simulink model "continuos_model"  (R2016b)
settings: Solver=VariableStepAuto  StartTime=0.0  StopTime=40  FixedStep=0.001  RelTol=1e-3
undefined symbols (not defined in the file or in its folder): DiscIntNeverNeededParam
libraries: dspsrcs4 x2
settings Model: Creator=Utente  LastModifiedBy=liana

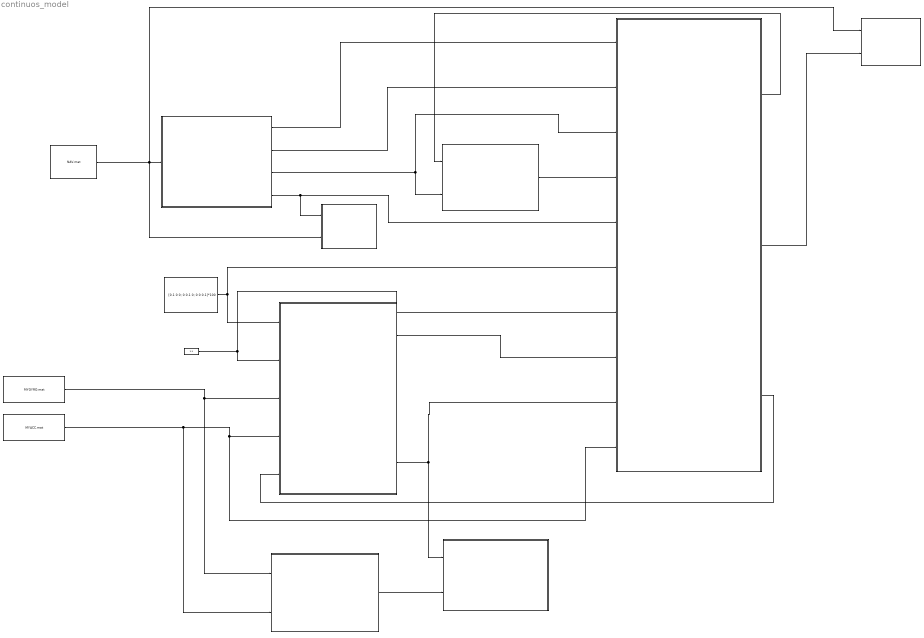
== system continuos_model ==
  Algebraic Transformation : Subsystem
  Attitude Observer : Subsystem
  Error position (AT) : Subsystem
  Error position (NLO) : Subsystem
  From File2 : FromFile  FileName=MYGYRO.mat
  From File3 : FromFile  FileName=MYACC.mat
  Gain computation : Subsystem
  Kp : Constant  Value=[0.1 0 0; 0 0.1 0; 0 0 0.1]*100  SampleTime=-1
  Mechanisation : Subsystem
  Translational Motion Observer : Subsystem
  Vehicle position in NED : FromFile  FileName=NAV.mat
  angles error : Subsystem
  sigma : Constant  Value=1.1  SampleTime=-1
  wires:
  From File2/1 -> Mechanisation/1(w_ib), Attitude Observer/3(w_ib)
  From File3/1 -> Mechanisation/2(f_b), Translational Motion Observer/10(f_b), Attitude Observer/4(f_b)
  Kp/1 -> Translational Motion Observer/6(K_p), Attitude Observer/1(Kp)
  sigma/1 -> Attitude Observer/2(sigma), Translational Motion Observer/7(sigma)
  Attitude Observer/1(J) -> Translational Motion Observer/8(J)
  Attitude Observer/3(R_nb_stim) -> Translational Motion Observer/9(R_nb_stim), angles error/1(R_nb_stim)
  Gain computation/1(K) -> Translational Motion Observer/4(K)
  Algebraic Transformation/3(C_dx) -> Translational Motion Observer/3(C_dx), Gain computation/2(C_dx)
  Translational Motion Observer/2(x_stim) -> Error position (NLO)/2(estimated)
  Vehicle position in NED/1 -> Error position (NLO)/1(true), Error position (AT)/2(true), Algebraic Transformation/1(p_n)
  Translational Motion Observer/3(f_n_stim) -> Attitude Observer/5(f_n_stim)
  Algebraic Transformation/4(x_at) -> Translational Motion Observer/5(Init), Error position (AT)/1(estimated)
  Mechanisation/1(R_nb) -> angles error/2(R_nb)
  Algebraic Transformation/1(p_n_i) -> Translational Motion Observer/1(p_n_i)
  Translational Motion Observer/1(C_dx_NLO) -> Gain computation/1(C_dx_NLO)
  Algebraic Transformation/2(delta) -> Translational Motion Observer/2(delta)

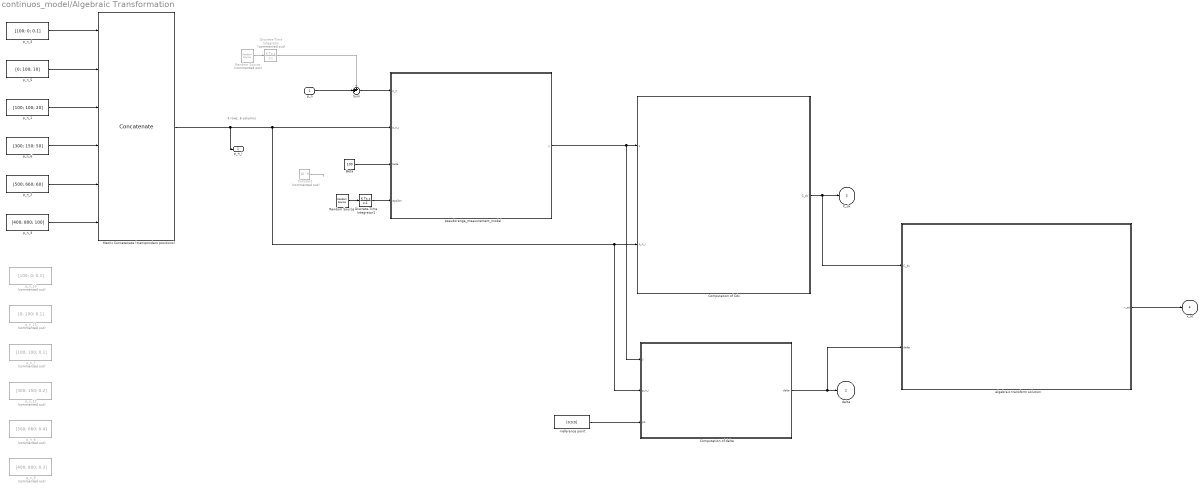
== system continuos_model/Algebraic Transformation ==
  note: 3 rows, 6 columns
  p_n : Inport
  Beta : Constant  Value=100  SampleTime=0.1
  Computation of Cdx : MATLAB Function  TreatAsAtomicUnit=on
  Computation of delta : MATLAB Function  TreatAsAtomicUnit=on
  Constant : Constant  Commented=on  Value=10^6
  Discrete-Time Integrator : DiscreteIntegrator  Commented=on  IntegratorMethod=Integration: Backward Euler  gainval=2  InitialConditionSetting=State (most efficient)  SampleTime=0.1  LimitOutput=on  UpperSaturationLimit=10  LowerSaturationLimit=-10  ICPrevOutput=DiscIntNeverNeededParam  ICPrevScaledInput=DiscIntNeverNeededParam
  Discrete-Time Integrator1 : DiscreteIntegrator  IntegratorMethod=Integration: Backward Euler  gainval=10  InitialConditionSetting=State (most efficient)  SampleTime=0.1  LimitOutput=on  UpperSaturationLimit=10  LowerSaturationLimit=-10  ICPrevOutput=DiscIntNeverNeededParam  ICPrevScaledInput=DiscIntNeverNeededParam
  Matrix Concatenate (transponders positions) : Concatenate  NumInputs=6  Mode=Multidimensional array  ConcatenateDimension=2
  Random Source : dspsrcs4/Random Source  Commented=on  SrcType=Gaussian  NormMethod=Ziggurat  CltLength=12  MinVal=0  MaxVal=1  MeanVal=[0;0;0]  VarVal=[1;1;1]*0.25  RepMode=Not repeatable  rawSeed=1  IsInherit=off  SampMode=Discrete  SampTime=0.1  SampFrame=1  DataType=Double  OutComplex=Real  OutputFrames=off
  Random Source1 : dspsrcs4/Random Source  SrcType=Gaussian  NormMethod=Ziggurat  CltLength=12  MinVal=0  MaxVal=1  MeanVal=0  VarVal=0.25  RepMode=Not repeatable  rawSeed=1  IsInherit=off  SampMode=Discrete  SampTime=0.1  SampFrame=1  DataType=Single  OutComplex=Real  OutputFrames=off
  Sum : Sum  Inputs=++|
  algebraic transform solution : MATLAB Function  TreatAsAtomicUnit=on
  p_n_1 : Constant  Value=[100; 100; 20]
  p_n_10 : Constant  Commented=on  Value=[100; 0; 0.1]
  p_n_11 : Constant  Commented=on  Value=[0; 100; 0.1]
  p_n_12 : Constant  Commented=on  Value=[300; 150; 0.2]
  p_n_2 : Constant  Value=[500; 660; 60]
  p_n_3 : Constant  Value=[400; 800; 100]
  p_n_4 : Constant  Value=[100; 0; 0.1]
  p_n_5 : Constant  Value=[0; 100; 10]
  p_n_6 : Constant  Value=[300; 150; 50]
  p_n_7 : Constant  Commented=on  Value=[100; 100; 0.1]
  p_n_8 : Constant  Commented=on  Value=[500; 660; 0.4]
  p_n_9 : Constant  Commented=on  Value=[400; 800; 0.3]
  pseudorange_measurement_model : MATLAB Function  TreatAsAtomicUnit=on
  rreference point : Constant  Value=[0;0;0]
  p_n_i : Outport
  delta : Outport  Port=2
  C_dx : Outport  Port=3
  x_at : Outport  Port=4
  wires:
  Beta/1 -> pseudorange_measurement_model/3(beta)
  Discrete-Time Integrator1/1 -> pseudorange_measurement_model/4(epsilon)
  pseudorange_measurement_model/1(y) -> Computation of delta/1(y), Computation of Cdx/1(y)
  Matrix Concatenate (transponders positions)/1 -> p_n_i/1, Computation of delta/2(p_n_i), Computation of Cdx/2(p_n_i), pseudorange_measurement_model/2(p_n_i)
  Computation of delta/1(delta) -> algebraic transform solution/2(delta), delta/1
  Computation of Cdx/1(C_dx) -> C_dx/1, algebraic transform solution/1(C_dx)
  rreference point/1 -> Computation of delta/3(p0)
  algebraic transform solution/1(x_at) -> x_at/1
  Sum/1 -> pseudorange_measurement_model/1(p_n)
  Discrete-Time Integrator/1 -> Sum/1
  Random Source/1 -> Discrete-Time Integrator/1
  p_n_4/1 -> Matrix Concatenate (transponders positions)/1
  p_n_5/1 -> Matrix Concatenate (transponders positions)/2
  p_n_1/1 -> Matrix Concatenate (transponders positions)/3
  p_n_6/1 -> Matrix Concatenate (transponders positions)/4
  p_n_2/1 -> Matrix Concatenate (transponders positions)/5
  p_n_3/1 -> Matrix Concatenate (transponders positions)/6
  p_n/1 -> Sum/2
  Random Source1/1 -> Discrete-Time Integrator1/1
  Constant/1 -> ?

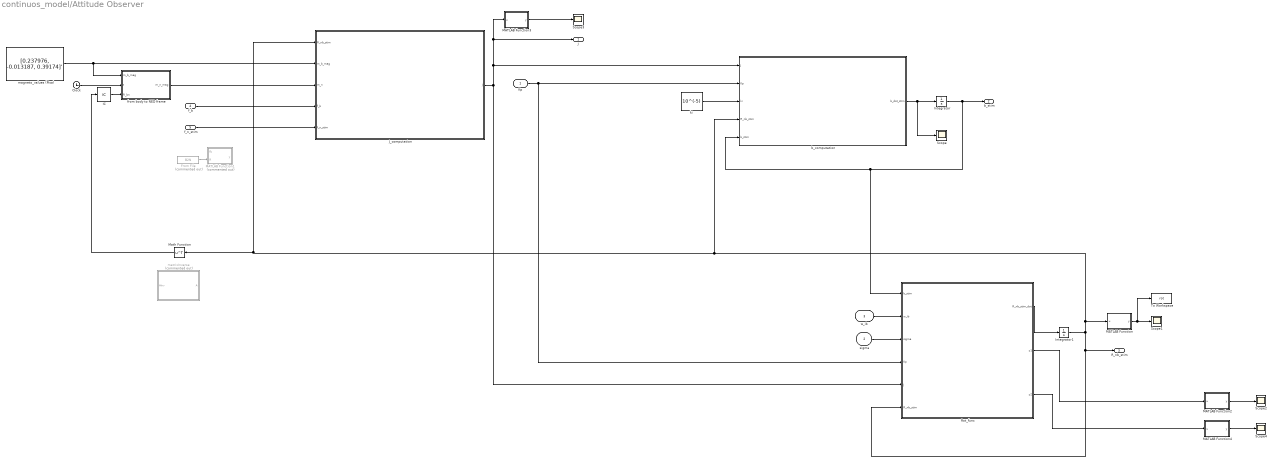
== system continuos_model/Attitude Observer ==
  Kp : Inport
  sigma : Inport  Port=2
  w_ib : Inport  Port=3
  f_b : Inport  Port=4
  f_n_stim : Inport  Port=5
  Clock : Clock
  From File : FromFile  Commented=on  FileName=B2N  SampleTime=0.01
  IC : InitialCondition  Value=eye(3)
  Integrator : Integrator
  Integrator1 : Integrator
  J_computation : Subsystem
  MATLAB Function : MATLAB Function  TreatAsAtomicUnit=on
  MATLAB Function1 : MATLAB Function  Commented=on  TreatAsAtomicUnit=on
  MATLAB Function2 : MATLAB Function  TreatAsAtomicUnit=on
  MATLAB Function3 : MATLAB Function  TreatAsAtomicUnit=on
  MATLAB Function4 : MATLAB Function  TreatAsAtomicUnit=on
  Math Function : Math  Operator=transpose  SaturateOnIntegerOverflow=on
  Rot_func : MATLAB Function  TreatAsAtomicUnit=on
  Scope{,1..4} (5 alike) : Scope
  To Workspace : ToWorkspace  VariableName=rot  SaveFormat=Timeseries  SampleTime=-1
  b_computation : MATLAB Function  TreatAsAtomicUnit=on
  from body to NED frame : MATLAB Function  TreatAsAtomicUnit=on
  ki : Constant  Value=10^(-5)  SampleTime=-1
  magneto_values (Pisa) : Constant  Value=[0.237976, -0.013187, 0.39174]'
  matrixInverse : MATLAB Function  Commented=on  TreatAsAtomicUnit=on
  J : Outport
  b_stim : Outport  Port=2
  R_nb_stim : Outport  Port=3
  wires:
  magneto_values (Pisa)/1 -> from body to NED frame/1(m_b_mag), J_computation/2(m_b_mag)
  from body to NED frame/1(m_n_mag) -> J_computation/3(m_n)
  f_b/1 -> J_computation/4(f_b)
  J_computation/1(J) -> MATLAB Function3/1(u), J/1, b_computation/1(J), Rot_func/5(J)
  Kp/1 -> Rot_func/4(Kp), b_computation/2(Kp)
  ki/1 -> b_computation/3(ki)
  sigma/1 -> Rot_func/3(sigma)
  w_ib/1 -> Rot_func/2(w_ib)
  Clock/1 -> from body to NED frame/2(t)
  b_computation/1(b_dot_stim) -> Scope/1, Integrator/1
  MATLAB Function/1(y) -> To Workspace/1, Scope1/1
  MATLAB Function3/1(y) -> Scope3/1
  Rot_func/1(R_nb_stim_dot) -> Integrator1/1
  Integrator/1 -> b_stim/1, Rot_func/1(b_stim), b_computation/5(b_stim)
  Integrator1/1 -> R_nb_stim/1, Rot_func/6(R_nb_stim), Math Function/1, J_computation/1(R_nb_stim), b_computation/4(R_nb_stim), MATLAB Function/1(u)
  f_n_stim/1 -> J_computation/5(f_n_stim)
  From File/1 -> MATLAB Function1/2(R)
  Math Function/1 -> IC/1
  IC/1 -> from body to NED frame/3(R_bn)
  Rot_func/2(y1) -> MATLAB Function2/1(u)
  Rot_func/3(y2) -> MATLAB Function4/1(u)
  MATLAB Function2/1(y) -> Scope2/1
  MATLAB Function4/1(y) -> Scope4/1

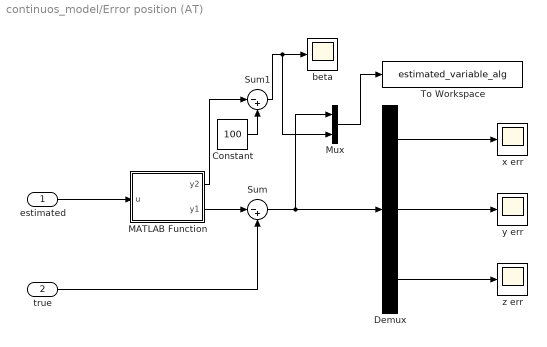
== system continuos_model/Error position (AT) ==
  estimated : Inport
  true : Inport  Port=2
  Constant : Constant  Value=100
  Demux : Demux  Outputs=3
  MATLAB Function : MATLAB Function  TreatAsAtomicUnit=on
  Mux : Mux  Inputs=2
  Sum : Sum  Inputs=|-+
  Sum1 : Sum  Inputs=|-+
  To Workspace : ToWorkspace  VariableName=estimated_variable_alg  SaveFormat=Timeseries  SampleTime=-1
  beta : Scope
  x err : Scope
  y err : Scope
  z err : Scope
  wires:
  MATLAB Function/2(y1) -> Sum/1
  true/1 -> Sum/2
  Sum/1 -> Mux/1, Demux/1
  Demux/1 -> x err/1
  Demux/2 -> y err/1
  Demux/3 -> z err/1
  estimated/1 -> MATLAB Function/1(u)
  Mux/1 -> To Workspace/1
  Sum1/1 -> Mux/2, beta/1
  MATLAB Function/1(y2) -> Sum1/1
  Constant/1 -> Sum1/2

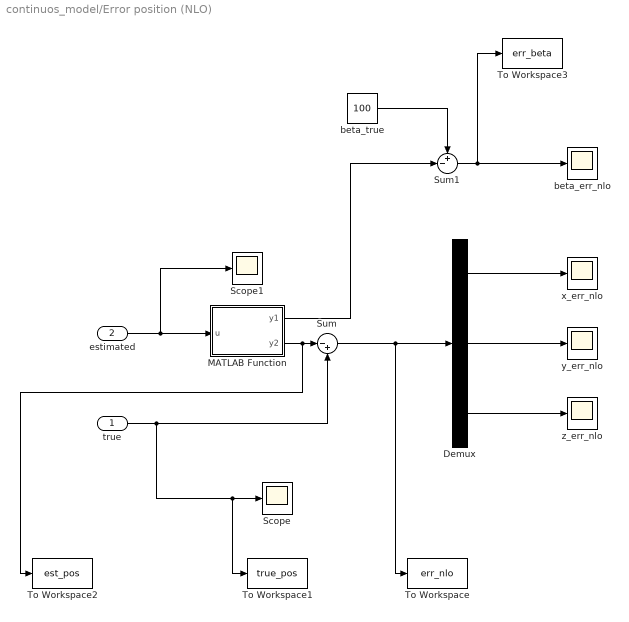
== system continuos_model/Error position (NLO) ==
  true : Inport
  estimated : Inport  Port=2
  Demux : Demux  Outputs=3
  MATLAB Function : MATLAB Function  TreatAsAtomicUnit=on
  Scope : Scope
  Scope1 : Scope
  Sum : Sum  Inputs=|-+
  Sum1 : Sum  Inputs=+-|
  To Workspace : ToWorkspace  VariableName=err_nlo  SaveFormat=Timeseries  SampleTime=-1
  To Workspace1 : ToWorkspace  VariableName=true_pos  SaveFormat=Timeseries  SampleTime=-1
  To Workspace2 : ToWorkspace  VariableName=est_pos  SaveFormat=Timeseries  SampleTime=-1
  To Workspace3 : ToWorkspace  VariableName=err_beta  SaveFormat=Timeseries  SampleTime=-1
  beta_err_nlo : Scope
  beta_true : Constant  Value=100
  x_err_nlo : Scope
  y_err_nlo : Scope
  z_err_nlo : Scope
  wires:
  estimated/1 -> Scope1/1, MATLAB Function/1(u)
  MATLAB Function/2(y2) -> To Workspace2/1, Sum/1
  true/1 -> To Workspace1/1, Scope/1, Sum/2
  Sum/1 -> To Workspace/1, Demux/1
  Demux/1 -> x_err_nlo/1
  Demux/2 -> y_err_nlo/1
  Demux/3 -> z_err_nlo/1
  MATLAB Function/1(y1) -> Sum1/2
  beta_true/1 -> Sum1/1
  Sum1/1 -> To Workspace3/1, beta_err_nlo/1

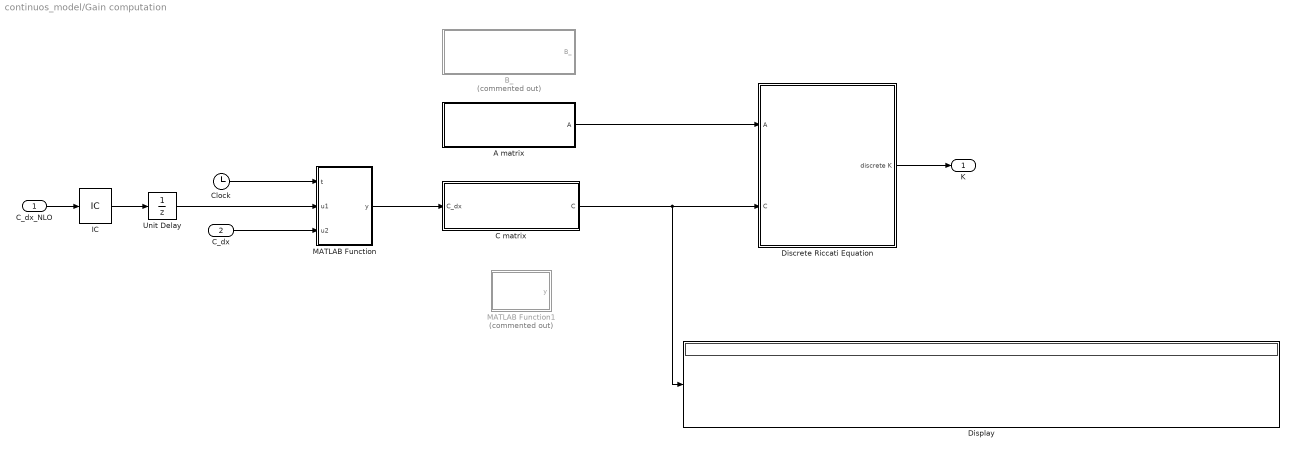
== system continuos_model/Gain computation ==
  C_dx_NLO : Inport
  C_dx : Inport  Port=2
  A matrix : MATLAB Function  TreatAsAtomicUnit=on
  B_ : MATLAB Function  Commented=on  TreatAsAtomicUnit=on
  C matrix : MATLAB Function  TreatAsAtomicUnit=on
  Clock : Clock
  Discrete Riccati Equation : Subsystem
  Display : Display
  IC : InitialCondition  Value=zeros(5,4)
  MATLAB Function : MATLAB Function  TreatAsAtomicUnit=on
  MATLAB Function1 : MATLAB Function  Commented=on  TreatAsAtomicUnit=on
  Unit Delay : UnitDelay  SampleTime=-1
  K : Outport
  wires:
  C matrix/1(C) -> Display/1, Discrete Riccati Equation/2(C)
  A matrix/1(A) -> Discrete Riccati Equation/1("A ")
  C_dx/1 -> MATLAB Function/3(u2)
  Discrete Riccati Equation/1(discrete K) -> K/1
  Clock/1 -> MATLAB Function/1(t)
  C_dx_NLO/1 -> IC/1
  MATLAB Function/1(y) -> C matrix/1(C_dx)
  IC/1 -> Unit Delay/1
  Unit Delay/1 -> MATLAB Function/2(u1)

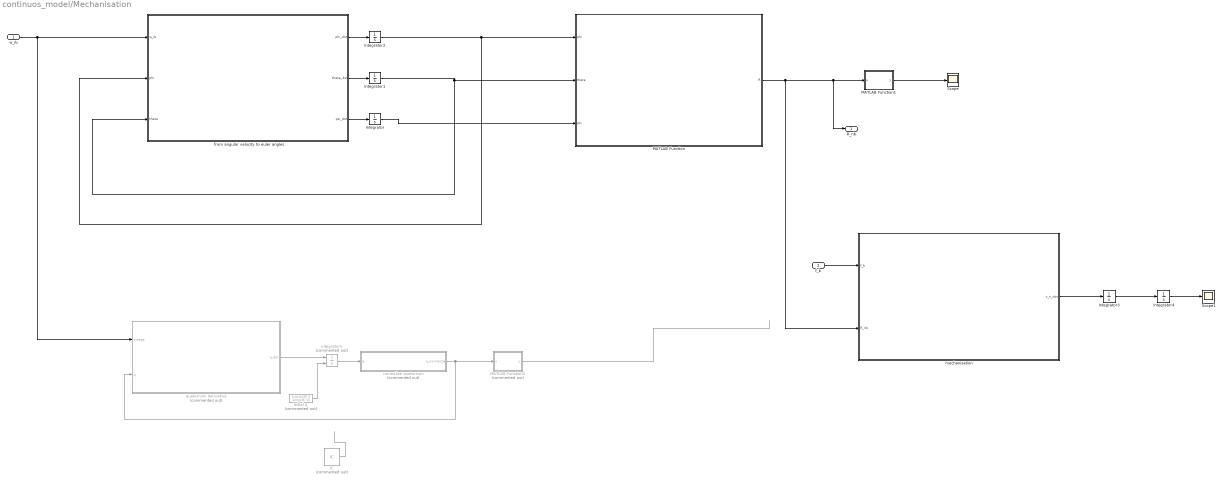
== system continuos_model/Mechanisation ==
  w_ib : Inport
  f_b : Inport  Port=2
  IC : InitialCondition  Commented=on  Value=[0 0 0 0]
  Initial q : Constant  Commented=on  Value=[cos(pi/8) 0 sin(pi/8) 0]  VectorParams1D=off
  Integrator{,1..4} (5 alike) : Integrator
  Integrator5 : Integrator  Commented=on  InitialConditionSource=external
  MATLAB Function : MATLAB Function  TreatAsAtomicUnit=on
  MATLAB Function1 : MATLAB Function  TreatAsAtomicUnit=on
  MATLAB Function2 : MATLAB Function  Commented=on  TreatAsAtomicUnit=on
  Scope : Scope
  Scope1 : Scope
  from angular velocity to euler angles : MATLAB Function  TreatAsAtomicUnit=on
  mechanisation : MATLAB Function  TreatAsAtomicUnit=on
  normalize quaternion : MATLAB Function  Commented=on  TreatAsAtomicUnit=on
  quaternion derivative : MATLAB Function  Commented=on  TreatAsAtomicUnit=on
  R_nb : Outport
  wires:
  from angular velocity to euler angles/1(phi_dot) -> Integrator2/1
  from angular velocity to euler angles/2(theta_dot) -> Integrator1/1
  from angular velocity to euler angles/3(psi_dot) -> Integrator/1
  MATLAB Function/1(R) -> mechanisation/2(R_nb), R_nb/1, MATLAB Function1/1(u)
  MATLAB Function1/1(y) -> Scope/1
  f_b/1 -> mechanisation/1(f_b)
  Integrator3/1 -> Integrator4/1
  Integrator4/1 -> Scope1/1
  Integrator1/1 -> from angular velocity to euler angles/3(theta), MATLAB Function/2(theta)
  Integrator/1 -> MATLAB Function/3(psi)
  Integrator2/1 -> from angular velocity to euler angles/2(phi), MATLAB Function/1(phi)
  quaternion derivative/1(q_dot) -> Integrator5/1
  Integrator5/1 -> normalize quaternion/1(q)
  w_ib/1 -> quaternion derivative/1(omega), from angular velocity to euler angles/1(w_ib)
  normalize quaternion/1(q_normalize) -> quaternion derivative/2(q), MATLAB Function2/1(u)
  IC/1 -> ?
  Initial q/1 -> Integrator5/2
  MATLAB Function2/1(y) -> ?
  mechanisation/1(v_n_dot) -> Integrator3/1

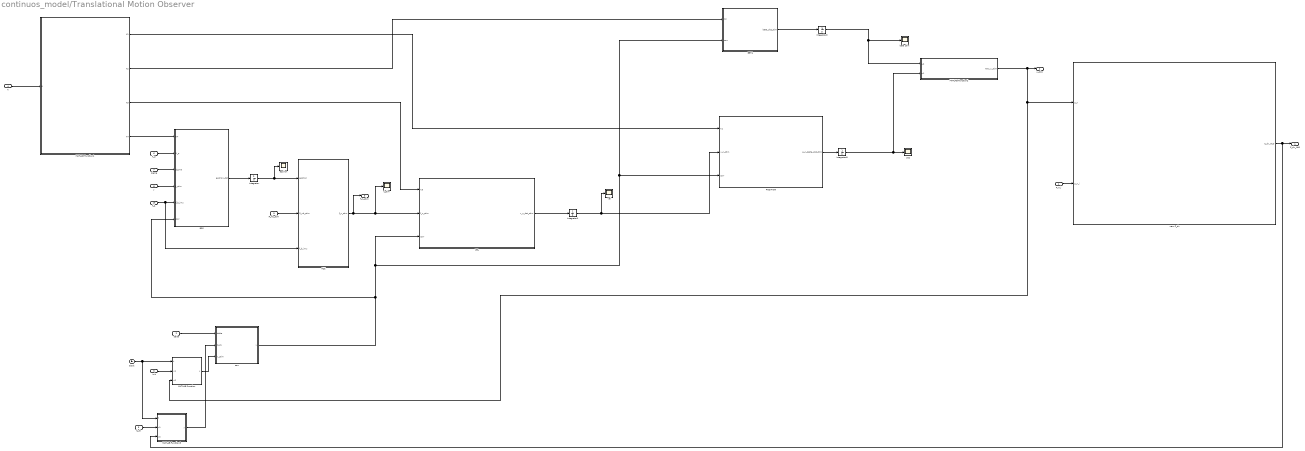
== system continuos_model/Translational Motion Observer ==
  p_n_i : Inport
  delta : Inport  Port=2
  C_dx : Inport  Port=3
  K : Inport  Port=4
  Init : Inport  Port=5
  K_p : Inport  Port=6
  sigma : Inport  Port=7
  J : Inport  Port=8
  R_nb_stim : Inport  Port=9
  f_b : Inport  Port=10
  ACC : MATLAB Function  TreatAsAtomicUnit=on
  BETA : MATLAB Function  TreatAsAtomicUnit=on
  Clock : Clock
      settings: Decimation=2
  EPS : MATLAB Function  TreatAsAtomicUnit=on
  Integrator : Integrator
  Integrator1 : Integrator
  Integrator2 : Integrator
  Integrator3 : Integrator  InitialCondition=[250;0;0]
  MATLAB Function : MATLAB Function  TreatAsAtomicUnit=on
  MATLAB Function1 : MATLAB Function  TreatAsAtomicUnit=on
  MATLAB Function2 : MATLAB Function  TreatAsAtomicUnit=on
  MATLAB Function3 : MATLAB Function  TreatAsAtomicUnit=on
  POSITION : MATLAB Function  TreatAsAtomicUnit=on
  VEL : MATLAB Function  TreatAsAtomicUnit=on
  beta stim : Scope
  corr : MATLAB Function  TreatAsAtomicUnit=on
  epsilon : Scope
  f_stim : Scope
  new C_dx : Subsystem
  pos : Scope
  vel : Scope
  C_dx_NLO : Outport
  x_stim : Outport  Port=2
  f_n_stim : Outport  Port=3
  wires:
  EPS/1(epsilon_dot) -> Integrator/1
  Integrator/1 -> epsilon/1, ACC/1(epsilon)
  MATLAB Function1/4(K4) -> EPS/1(K4)
  MATLAB Function1/1(K1) -> POSITION/1(K1)
  MATLAB Function1/3(K3) -> VEL/1(K3)
  MATLAB Function1/2(K2) -> BETA/1(K2)
  K/1 -> MATLAB Function1/1(K)
  K_p/1 -> EPS/2(K_p)
  sigma/1 -> EPS/3(sigma)
  J/1 -> EPS/4(J_stim)
  f_b/1 -> ACC/3(f_b_imu), EPS/5(f_b_imu)
  R_nb_stim/1 -> ACC/2(R_nb_stim)
  C_dx/1 -> MATLAB Function3/2(u1)
  delta/1 -> corr/1(delta)
  Init/1 -> MATLAB Function/2(u1)
  MATLAB Function/1(y) -> corr/3(x_stim)
  Clock/1 -> MATLAB Function3/1(t), MATLAB Function/1(t)
  ACC/1(f_n_stim) -> f_n_stim/1, VEL/2(f_n_stim), f_stim/1
  VEL/1(v_n_dot_stim) -> Integrator1/1
  BETA/1(beta_dot_stim) -> Integrator2/1
  POSITION/1(p_n_delta_dot_stim) -> Integrator3/1
  new C_dx/1(C_dx_NLO) -> MATLAB Function3/3(u2), C_dx_NLO/1
  MATLAB Function3/1(y) -> corr/2(C_dx)
  corr/1(y) -> BETA/2(corr), POSITION/3(corr), VEL/3(corr), EPS/6(corr)
  p_n_i/1 -> new C_dx/2(p_n_i)
  Integrator1/1 -> vel/1, POSITION/2(v_n_stim)
  Integrator3/1 -> MATLAB Function2/2(u1), pos/1
  Integrator2/1 -> beta stim/1, MATLAB Function2/1(u2)
  MATLAB Function2/1(new_x_stim) -> x_stim/1, new C_dx/1(p_n), MATLAB Function/3(u2)

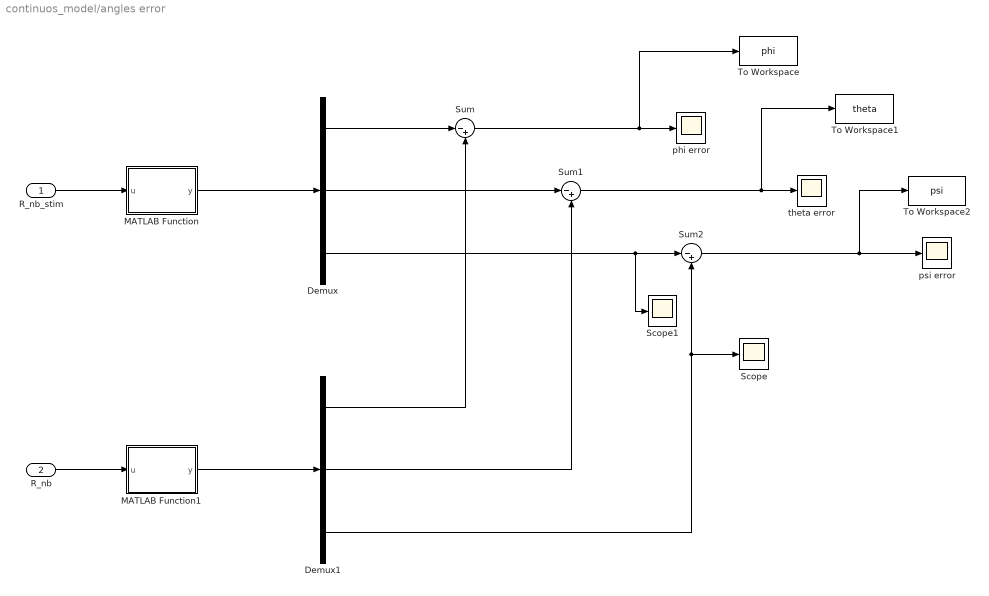
== system continuos_model/angles error ==
  R_nb_stim : Inport
  R_nb : Inport  Port=2
  Demux : Demux  Outputs=3
  Demux1 : Demux  Outputs=3
  MATLAB Function : MATLAB Function  TreatAsAtomicUnit=on
  MATLAB Function1 : MATLAB Function  TreatAsAtomicUnit=on
  Scope : Scope
  Scope1 : Scope
  Sum : Sum  Inputs=|-+
  Sum1 : Sum  Inputs=|-+
  Sum2 : Sum  Inputs=|-+
  To Workspace : ToWorkspace  VariableName=phi  SaveFormat=Timeseries  SampleTime=-1
  To Workspace1 : ToWorkspace  VariableName=theta  SaveFormat=Timeseries  SampleTime=-1
  To Workspace2 : ToWorkspace  VariableName=psi  SaveFormat=Timeseries  SampleTime=-1
  phi error : Scope
  psi error : Scope
  theta error : Scope
  wires:
  R_nb_stim/1 -> MATLAB Function/1(u)
  R_nb/1 -> MATLAB Function1/1(u)
  MATLAB Function/1(y) -> Demux/1
  MATLAB Function1/1(y) -> Demux1/1
  Demux/1 -> Sum/1
  Demux/2 -> Sum1/1
  Demux/3 -> Scope1/1, Sum2/1
  Demux1/1 -> Sum/2
  Demux1/2 -> Sum1/2
  Demux1/3 -> Scope/1, Sum2/2
  Sum/1 -> To Workspace/1, phi error/1
  Sum1/1 -> To Workspace1/1, theta error/1
  Sum2/1 -> To Workspace2/1, psi error/1

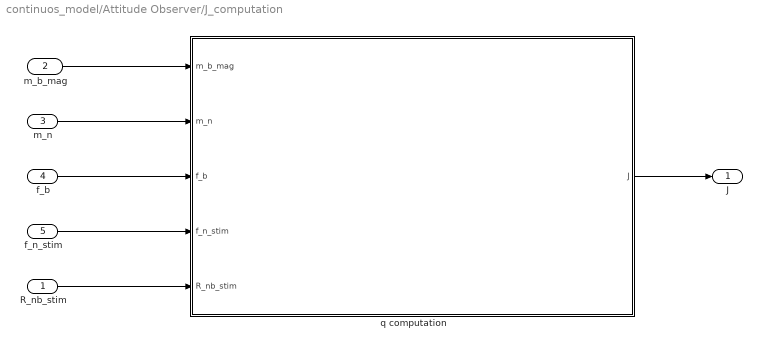
== system continuos_model/Attitude Observer/J_computation ==
  R_nb_stim : Inport
  m_b_mag : Inport  Port=2
  m_n : Inport  Port=3
  f_b : Inport  Port=4
  f_n_stim : Inport  Port=5  PortDimensions=[3,1]
  q computation : MATLAB Function  TreatAsAtomicUnit=on
  J : Outport
  wires:
  m_n/1 -> q computation/2(m_n)
  f_n_stim/1 -> q computation/4(f_n_stim)
  m_b_mag/1 -> q computation/1(m_b_mag)
  f_b/1 -> q computation/3(f_b)
  q computation/1(J) -> J/1
  R_nb_stim/1 -> q computation/5(R_nb_stim)

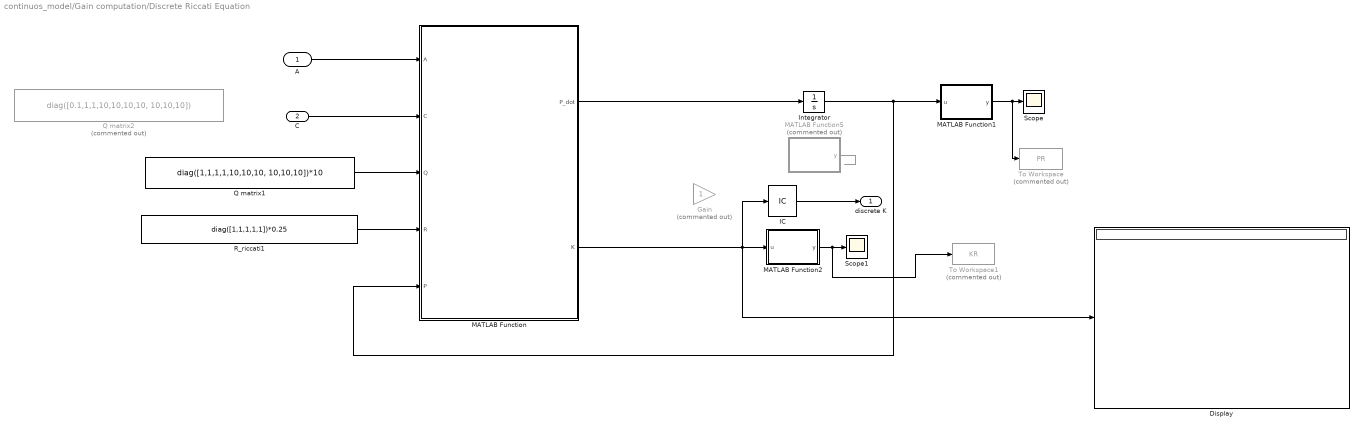
== system continuos_model/Gain computation/Discrete Riccati Equation ==
  "A " : Inport
  C : Inport  Port=2
  Display : Display
  Gain : Gain  Commented=on
  IC : InitialCondition  Value=0
  Integrator : Integrator  InitialCondition=eye(10)*0.1  AbsoluteTolerance=0.00000001
  MATLAB Function : MATLAB Function  TreatAsAtomicUnit=on
  MATLAB Function1 : MATLAB Function  TreatAsAtomicUnit=on
  MATLAB Function2 : MATLAB Function  TreatAsAtomicUnit=on
  MATLAB Function5 : MATLAB Function  Commented=on  TreatAsAtomicUnit=on
  Q matrix1 : Constant  Value=diag([1,1,1,1,10,10,10, 10,10,10])*10  VectorParams1D=off  SampleTime=-1
  Q matrix2 : Constant  Commented=on  Value=diag([0.1,1,1,10,10,10,10, 10,10,10])  VectorParams1D=off  SampleTime=-1
  R_riccati1 : Constant  Value=diag([1,1,1,1,1])*0.25  VectorParams1D=off  SampleTime=-1
  Scope : Scope
  Scope1 : Scope
  To Workspace : ToWorkspace  Commented=on  VariableName=PR  SaveFormat=Timeseries  SampleTime=-1
  To Workspace1 : ToWorkspace  Commented=on  VariableName=KR  SaveFormat=Timeseries  SampleTime=-1
  discrete K : Outport
  wires:
  C/1 -> MATLAB Function/2(C)
  Q matrix1/1 -> MATLAB Function/3(Q)
  R_riccati1/1 -> MATLAB Function/4(R)
  Integrator/1 -> MATLAB Function1/1(u), MATLAB Function/5(P)
  MATLAB Function1/1(y) -> To Workspace/1, Scope/1
  MATLAB Function2/1(y) -> To Workspace1/1, Scope1/1
  MATLAB Function/1(P_dot) -> Integrator/1
  MATLAB Function5/1(y) -> ?
  "A "/1 -> MATLAB Function/1(A)
  MATLAB Function/2(K) -> IC/1, Display/1, MATLAB Function2/1(u)
  IC/1 -> discrete K/1

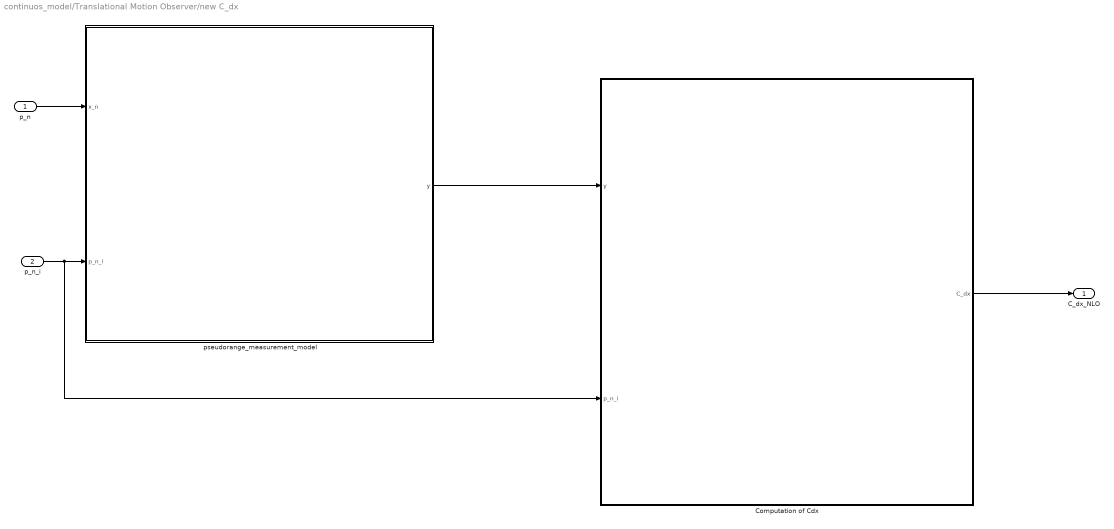
== system continuos_model/Translational Motion Observer/new C_dx ==
  p_n : Inport
  p_n_i : Inport  Port=2
  Computation of Cdx : MATLAB Function  TreatAsAtomicUnit=on
  pseudorange_measurement_model : MATLAB Function  TreatAsAtomicUnit=on
  C_dx_NLO : Outport
  wires:
  p_n_i/1 -> Computation of Cdx/2(p_n_i), pseudorange_measurement_model/2(p_n_i)
  pseudorange_measurement_model/1(y) -> Computation of Cdx/1(y)
  Computation of Cdx/1(C_dx) -> C_dx_NLO/1
  p_n/1 -> pseudorange_measurement_model/1(x_n)

== matlab function continuos_model/Attitude Observer/J_computation/q computation ==
  data: m_b_mag input; m_n input; f_b input; f_n_stim input size=3; J output; R_nb_stim input size=[3,3]
function J  = qEfunc(m_b_mag, m_n, f_b, f_n_stim, R_nb_stim)

g_n = [0.1 0.1 0.1]';   % gravity compensated

q1_b = m_b_mag/norm(m_b_mag,2);
q2_b = f_b/norm(g_n,2);

q1_n = m_n/norm(m_n,2);
q2_n = f_n_stim/norm(g_n,2);

E_b = [q1_b, skew(q1_b)*q2_b, (skew(q1_b)*skew(q1_b))*q2_b];
E_n = [q1_n, skew(q1_n)*q2_n, (skew(q1_n)*skew(q1_n))*q2_n];

J = (E_n - R_nb_stim * E_b) * (E_b');

end

== matlab function continuos_model/Error position (AT)/MATLAB Function ==
  data: y2 output; u input; y1 output
function [y2,y1] = fcn(u)

y1 = u(1:3,1);
y2 = u(4,1);

== matlab function continuos_model/Translational Motion Observer/MATLAB Function ==
  data: t input; y output; u1 input; u2 input
function y = fcn(t,u1,u2)

if t == 0
    y = u1;
else
    y = u2;
end

== matlab function continuos_model/Error position (NLO)/MATLAB Function ==
  data: u input; y1 output; y2 output
function [y1,y2] = fcn(u)

y1 = u(4,1);
y2 = u(1:3,1);

== matlab function continuos_model/angles error/MATLAB Function ==
  data: u input; y output
function y = fcn(u)

y = rotm2eul(u,'ZYX');

== matlab function continuos_model/angles error/MATLAB Function1 ==
  data: u input; y output
function y = fcn(u)

y = rotm2eul(u,'ZYX');

== matlab function continuos_model/Attitude Observer/b_computation ==
  data: J input; b_dot_stim output size=3; Kp input; ki input; R_nb_stim input; b_stim input
function b_dot_stim  = b_dot_stim_func(J, Kp, ki, R_nb_stim, b_stim)

SAT = sat(R_nb_stim)';

PA = pa( SAT * Kp * J);

VEX = vexfunc(PA);

b_dot_stim = Proj(b_stim , -ki * VEX);

end

== matlab function continuos_model/Translational Motion Observer/new C_dx/Computation of Cdx ==
  data: y input; p_n_i input; C_dx output size=[5,4]
function C_dx  = C_dx_func(y,p_n_i)

    [row,col] = size(p_n_i);
    [row_,col_] = size(y);

    % taking last transponder position
    p_m = p_n_i(:,col);
    
    % col is the number of transponders
    
    % taking last pseudorange measurement
    y_m = y(row_);
    
    %row vector, 3 stands for x,y,z
    p_ = zeros(col-1,3); 
    y_ = zeros(col-1,1);
    
    for i = 1:1:(col-1)
    
        p_(i,:) = (p_m - p_n_i(:,i))';
        
        y_(i,1) = y(i,1) - y_m;
        
    end
    
    C_dx = [p_, y_];

end

== matlab function continuos_model/Algebraic Transformation/Computation of Cdx ==
  data: y input; p_n_i input; C_dx output size=[5,4]
function C_dx  = C_dx_func(y,p_n_i)

    [row,col] = size(p_n_i);
    [row_,col_] = size(y);

    % taking last transponder position
    p_m = p_n_i(:,col);
    
    % col is the number of transponders
    
    % taking last pseudorange measurement
    y_m = y(row_);
    
    %row vector, 3 stands for x,y,z
    p_ = zeros(col-1,3); 
    y_ = zeros(col-1,1);
    
    for i = 1:1:(col-1)
    
        p_(i,:) = (p_m - p_n_i(:,i))';
        
        y_(i,1) = y(i,1) - y_m;
        
    end
    
    C_dx = [p_, y_];

end

== matlab function continuos_model/Algebraic Transformation/Computation of delta ==
  data: y input; delta output size=5; p_n_i input; p0 input
function delta = delta_func(y, p_n_i, p0)
    
    % col is the number of transponders
    [row,col] = size(p_n_i);
    %[row_,col_] = size(y);
    
    % line of sight between transponders and reference point
    p_los = zeros(row,col);
    
    for i = 1:1:col
       p_los(:,i) = p_n_i(:,i) - p0;
    end
    
    % useful variable
    z = zeros(col,1);
    
    for i = 1:1:col
        z(i,1)= ( (y(i,1)^2) - norm(p_los(:,i),2)^2 );
    end
    
    % computing delta
    delta = zeros(col-1,1);
    % last value of z
    z_m = z(col,1);
    
    for i=1:1:(col-1)
        delta(i,1) = z(i,1) - z_m;
    end
    
end

== matlab function continuos_model/Translational Motion Observer/new C_dx/pseudorange_measurement_model ==
  data: x_n input; y output size=[6,1]; p_n_i input
function y = pseudorange_mea_model(x_n, p_n_i)
  
  [r,c] = size(p_n_i);
  
  p_n = x_n(1:3,1);
  beta = x_n(4,1);
  
  y = zeros(c,1);

  for i=1:1:c
      
      rho = norm(p_n - p_n_i(:,i),2);   % eq. 7
      
      y(i,1) = rho + beta;      % eq. 8 

  end
      
end

== matlab function continuos_model/Gain computation/MATLAB Function ==
  data: t input; y output; u1 input; u2 input
function y = fcn(t,u1,u2)

if t==0
    y = u2;
else
    y = u1;
end

== matlab function continuos_model/Translational Motion Observer/MATLAB Function3 ==
  data: t input; y output; u1 input; u2 input
function y = fcn(t,u1,u2)

if t == 0
    y = u1;
else
    y = u2;
end

== matlab function continuos_model/Attitude Observer/Rot_func ==
  data: b_stim input; R_nb_stim_dot output; w_ib input; sigma input; Kp input; J input; R_nb_stim input; y1 output; y2 output
function [R_nb_stim_dot,y1,y2]  = rot_func(b_stim,w_ib,sigma,Kp,J,R_nb_stim) 

Skew = skew(w_ib - b_stim);

R_nb_stim_dot = R_nb_stim * Skew + sigma * Kp * J;

y1 = R_nb_stim * Skew;
y2 = sigma * Kp * J;

== matlab function continuos_model/Attitude Observer/MATLAB Function2 ==
  data: u input; y output
function y = fcn(u)

y = rotm2eul(u,'ZYX');

== matlab function continuos_model/Attitude Observer/MATLAB Function4 ==
  data: u input; y output
function y = fcn(u)

y = rotm2eul(u,'ZYX');

== matlab function continuos_model/Gain computation/A matrix ==
  data: A output
function A = A()

 A = zeros(10);

 A(1:3,5:7) = eye(3);
 A(5:7,8:10) = eye(3);
 
end

== matlab function continuos_model/Gain computation/C matrix ==
  data: C output; C_dx input
function C = Cfunc(C_dx)

   row = size(C_dx,1); 

   C1 = zeros(row,6);

 C = [2*C_dx C1];
 
 
end

== matlab function continuos_model/Gain computation/B_ ==
  data: B_ output
function B_ = B()

 B_ = zeros(10,3);

 B_(8:10,1:3) = eye(3);
end

== matlab function continuos_model/Algebraic Transformation/pseudorange_measurement_model ==
  data: p_n input; y output size=[6,1]; p_n_i input; beta input; epsilon input
function y = pseudorange_mea_model(p_n, p_n_i, beta, epsilon)
  
  [r,c] = size(p_n_i);
  
  y = zeros(c,1);

  for i=1:1:c
      
      rho = norm(p_n - p_n_i(:,i),2);   % eq. 7
      
      y(i,1) = rho + beta + epsilon;      % eq. 8 

  end
      
end

== matlab function continuos_model/Attitude Observer/from body to NED frame ==
  data: m_b_mag input; t input; R_bn input; m_n_mag output
function m_n_mag = b2n(m_b_mag, t, R_bn)

% m_n_mag and m_b_mag are 3x1

% if t==0
%     R_bn = eye(3);
% end

m_n_mag = R_bn * m_b_mag;

== matlab function continuos_model/Attitude Observer/matrixInverse ==
  data: A input; AInv output
function AInv  = matrixInverse(A)

% AInv = inv(A);

% inverse by singular value decomposition


[n,m] = size(A);

% % % U = zeros(n,n);
% % % V = zeros(n,n);
% % % S = zeros(n,n);

[U,S,V] = svd(A);

pos = 0;

% % % maximun admissible condition number
csi = 10^3;

for i=n:-1:1
    if( S(1,1)/S(i,i) > csi)
        S(i,i) = 0;
        pos = i; % keeps the last eliminated singular value
    end
end

tempS = S(1:pos-1,1:pos-1); %take the non-zero set
tempS = inv(tempS);
S(1:pos-1,1:pos-1) = tempS(1:pos-1,1:pos-1); % now S is the inverse matrix
AInv = V * S * U';

end

== matlab function continuos_model/Attitude Observer/MATLAB Function1 ==
  data: fb input; y output; R input
function y = fcn(fb,R)

y = R*fb;

== matlab function continuos_model/Gain computation/MATLAB Function1 ==
  data: y output
function y = fcn()

 y =    1.0e+03 * [    -1.0000   -0.1800    0.0180    1.0125         0         0         0         0         0         0;
                       -0.4000   -0.3200    0.0160    0.4622         0         0         0         0         0         0;
                       -2.4000   -0.3600    0.0120    2.4239         0         0         0         0         0         0;
                       -1.3000   -0.4600   -0.0020    1.3634         0         0         0         0         0         0;
                       -0.9000   -0.2600    0.0040    0.9280         0         0         0         0         0         0];

== matlab function continuos_model/Mechanisation/normalize quaternion ==
  data: q_normalize output; q input
function q_normalize = quatEstNormalized(q)
% This block normalized the estimated quaternion 

q_normalize = quatnormalize(q);

== matlab function continuos_model/Mechanisation/quaternion derivative ==
  data: omega input; q_dot output; q input
function q_dot = quatDotEst(omega, q)
% This block estimates the quaternion derivative 

omega = omega';

q_dot = zeros(1,4);

q_dot(1) = -0.5*dot(q(2:4),omega);
q_dot(2:4) = 0.5*(cross(q(2:4),omega) + omega*q(1));

== matlab function continuos_model/Mechanisation/MATLAB Function2 ==
  data: u input; y output
function y = fcn(u)

y = quat2rotm(u);

== matlab function continuos_model/Mechanisation/from angular velocity to euler angles ==
  data: w_ib input; phi input; theta input; phi_dot output; theta_dot output; psi_dot output
function [phi_dot, theta_dot, psi_dot] = w2doteuler(w_ib, phi, theta)


D = zeros(3,3);
D(1,1) = 1;
D(1,2) = sin(phi)*tan(theta);
D(1,3) = cos(phi)*tan(theta);

D(2,2) = cos(phi);
D(2,3) = -sin(phi);

D(3,2) = sin(phi)/cos(theta);
D(3,3) = cos(phi)/cos(theta); 


% D = [ 1    sin(phi)*tan(theta)     cos(phi)*tan(theta);
%       0        cos(phi)                - sin(phi);
%       0    sin(phi)/cos(theta)     cos(phi)/cos(theta)]; 

phi_dot = D(1,:) * w_ib;
theta_dot = D(2,:) * w_ib;
psi_dot = D(3,:) * w_ib;

end

== matlab function continuos_model/Mechanisation/MATLAB Function ==
  data: phi input; R output; theta input; psi input
function R = eul2R(phi, theta, psi)

angles = [phi theta psi];

R = eul2rotm(angles,'ZYX');

end

== matlab function continuos_model/Mechanisation/MATLAB Function1 ==
  data: u input; y output
function y = fcn(u)

y = norm(u);

== matlab function continuos_model/Mechanisation/mechanisation ==
  data: f_b input; v_n_dot output; R_nb input
function v_n_dot  = mechanisation(f_b, R_nb)

g_n = [0.1 0.1 0.1]';   % gravity compensated

v_n_dot = R_nb * f_b + g_n;

end

== matlab function continuos_model/Attitude Observer/MATLAB Function ==
  data: u input; y output
function y = fcn(u)

% ckecking if norm == 1

y = norm(u,2);

== matlab function continuos_model/Attitude Observer/MATLAB Function3 ==
  data: u input; y output
function y = fcn(u)

y = norm(u);

== matlab function continuos_model/Algebraic Transformation/algebraic transform solution ==
  data: C_dx input; x_at output; delta input size=[5,1]
function x_at = solAT(C_dx, delta)

% inverse

pC_dx = pinv(C_dx);

x_at = pC_dx * (delta / 2);


% % % % [n,m] = size(C_dx);
% % % % 
% % % % % U = zeros(n,n);
% % % % % V = zeros(n,n);
% % % % % S = zeros(n,n);
% % % % 
% % % % [U,S,V] = svd(C_dx);
% % % % 
% % % % pos = 0;
% % % % 
% % % % % maximun admissible condition number
% % % % csi = 10^3;
% % % % 
% % % % for i=m:-1:1
% % % %     if( S(1,1)/S(i,i) > csi)
% % % %         S(i,i) = 0;
% % % %         pos = i; % keeps the last eliminated singular value
% % % %     end
% % % % end
% % % % 
% % % % % rebuild C_dx matrix
% % % % C_dx = U * S * V';
% % % % 
% % % % % % tempS = S(1:pos-1,1:pos-1); %take the non-zero set
% % % % % % tempS = inv(tempS);
% % % % % % S(1:pos-1,1:pos-1) = tempS(1:pos-1,1:pos-1); % now S is the inverse matrix
% % % % % % AInv = V * S * U';
% % % % 
% % % % 
% % % % % this solution is described in the Appendix
% % % % % and it is true only for m >= 5




end

== matlab function continuos_model/Gain computation/Discrete Riccati Equation/MATLAB Function ==
  data: A input; P_dot output; C input; Q input; R input; P input; K output
function [P_dot,K] = fcn(A,C,Q,R,P)

P_dot = A'*P + P*A - P*C'*inv(R)*C*P + Q;

K = P*C'*inv(R);

== matlab function continuos_model/Translational Motion Observer/MATLAB Function1 ==
  data: K input; K1 output; K2 output; K3 output; K4 output
function [K1,K2,K3,K4] = divK(K)

 K1 = K(1:3,:); 
 K2 = K(4,:);
 K3 = K(5:7,:);
 K4 = K(8:10,:);
 
end

== matlab function continuos_model/Translational Motion Observer/EPS ==
  data: K4 input; epsilon_dot output; K_p input; sigma input; J_stim input; f_b_imu input; corr input
function epsilon_dot = accel(K4,K_p, sigma, J_stim, f_b_imu, corr)

epsilon_dot   = -sigma * K_p * J_stim * f_b_imu + K4 * (corr); % eq 17

end

== matlab function continuos_model/Translational Motion Observer/ACC ==
  data: epsilon input; R_nb_stim input; f_n_stim output; f_b_imu input
function f_n_stim = fcn(epsilon,R_nb_stim, f_b_imu)

f_n_stim = R_nb_stim * f_b_imu + epsilon ;

end

== matlab function continuos_model/Translational Motion Observer/VEL ==
  data: K3 input; f_n_stim input; v_n_dot_stim output; corr input
function v_n_dot_stim = fcn(K3,f_n_stim, corr)

g_n = [0.1;0.1;0.1];

v_n_dot_stim = f_n_stim + g_n + K3*(corr);

== matlab function continuos_model/Translational Motion Observer/POSITION ==
  data: K1 input; v_n_stim input; p_n_delta_dot_stim output; corr input
function p_n_delta_dot_stim  = fcn(K1,v_n_stim,corr)

p_n_delta_dot_stim = v_n_stim + K1 * (corr);       % eq 14

end

== matlab function continuos_model/Translational Motion Observer/BETA ==
  data: K2 input; beta_dot_stim output; corr input
function beta_dot_stim = fcn(K2,corr)

beta_dot_stim = K2 * (corr);

== matlab function continuos_model/Translational Motion Observer/MATLAB Function2 ==
  data: u2 input; u1 input; new_x_stim output size=[4,1]
function new_x_stim = fcn(u2,u1)

new_x_stim = zeros(4,1);

new_x_stim(1:3,1) = u1;
new_x_stim(4,1) = u2;

end

== matlab function continuos_model/Translational Motion Observer/corr ==
  data: delta input; y output size=[5,1]; C_dx input; x_stim input size=[4,1]
function y = fcn(delta, C_dx, x_stim)

% delta and C_dx_x comes from algebraic transformation
% the first x_stim too, then by NLO

y = (delta - 2*C_dx*x_stim) ;

== matlab function continuos_model/Gain computation/Discrete Riccati Equation/MATLAB Function1 ==
  data: u input; y output
function y = fcn(u)

y = norm(u,2);

== matlab function continuos_model/Gain computation/Discrete Riccati Equation/MATLAB Function2 ==
  data: u input; y output
function y = fcn(u)

y = norm(u,inf);

== matlab function continuos_model/Gain computation/Discrete Riccati Equation/MATLAB Function5 ==
  data: y output
function y = fcn()

% gain computed by dare

% y =   [      0         0         0         0         0;
%          0         0         0         0         0;
%          0         0         0         0         0;
%          0         0         0         0         0;
%     0.0041   -0.0073    0.0034   -0.0061   -0.0027;
%     0.0019   -0.0042    0.0025   -0.0039   -0.0014;
%     0.0064    0.0627   -0.0137   -0.0051    0.0087;
%          0         0         0         0         0;
%          0         0         0         0         0;
%          0         0         0         0         0];


   y =  [     0         0         0         0         0;
             0         0         0         0         0;
             0         0         0         0         0;
             0         0         0         0         0;
        0.0041   -0.0073    0.0034   -0.0062   -0.0026;
        0.0019   -0.0042    0.0025   -0.0039   -0.0014;
        0.0060    0.0636   -0.0139   -0.0043    0.0085;
             0         0         0         0         0;
             0         0         0         0         0;
             0         0         0         0         0];




% y = [338.0836 -251.3072 -528.1877 -619.4670 -399.7782;
%  -535.8536   27.3842  454.0360 -710.6385   30.9063;
%   191.9185  938.7820 -163.0274 -207.9268  109.7480;
%   737.8810  -69.3387  656.6684 -138.8543   15.1638;
%     0.0037   -0.0066    0.0031   -0.0056   -0.0027;
%     0.0018   -0.0039    0.0024   -0.0036   -0.0015;
%     0.0076    0.0605   -0.0128   -0.0068    0.0087;
%     0.0000   -0.0000    0.0000   -0.0000   -0.0000;
%     0.0000   -0.0000    0.0000   -0.0000   -0.0000;
%     0.0000    0.0000   -0.0000   -0.0000    0.0000];
